simulink model "SoftABS_Hyd_RTW"  (R2022a)
settings: Solver=ode1  StartTime=0.0  StopTime=inf  FixedStep=0.001  RelTol=1e-3
PreLoadFcn:
  | vehicle = 'Car'; if ~length(which('cmcmd')), cmenv; end
  | SoftABS_Hyd_RTW_bus
  | SoftABS_Hyd_RTW_params
InitFcn:
  | vehicle = 'Car'; if ~length(which('cmcmd')), cmenv; end
  | SoftABS_Hyd_RTW_bus
  | SoftABS_Hyd_RTW_params
undefined symbols (not defined in the file or in its folder): f_ax, f_slip, sku_HA, sku_off_HA, sku_off_VA, sku_VA, t_Sensor, v_min, Valve_LUTin_HA, Valve_LUTin_VA, ValveIn_LUTout_HA, ValveIn_LUTout_VA, ValveOut_LUTout_HA, ValveOut_LUTout_VA
libraries: CarMaker4SL x23
Description:
  | CarMaker Plug-in Model Target
settings Model: ModifiedByFormat=IPG  Creator=IPG  LastModifiedBy=IPG
settings SolverCC: AlgebraicLoopSolver=TrustRegion
settings DataIOCC: LimitDataPoints=on  SaveFormat=Array  SignalLoggingSaveFormat=ModelDataLogs  ReturnWorkspaceOutputs=off
settings OptimizationCC: ExpressionDepthLimit=2147483647  LifeSpan=inf
settings DebuggingCC: UnderspecifiedInitializationDetection=Classic  MergeDetectMultiDrivingBlocksExec=none  FcnCallInpInsideContextMsg=warning  UnconnectedInputMsg=warning  UnconnectedOutputMsg=warning  UnconnectedLineMsg=warning  StateNameClashWarn=warning  SFUnexpectedBacktrackingDiag=warning  SFNoUnconditionalDefaultTransitionDiag=warning  SFMachineParentedDataDiag=warning  ArithmeticOperatorsInVariantConditions=warning
settings HardwareCC: ProdBitPerPointer=32  ProdBitPerSizeT=32  ProdBitPerPtrDiffT=32  ProdLargestAtomicFloat=None  ProdIntDivRoundTo=Undefined  ProdEndianess=Unspecified  ProdWordSize=32  ProdHWDeviceType=32-bit Generic  TargetHWDeviceType=32-bit Generic  ProdEqTarget=off
settings ModelReferenceCC: PropagateSignalLabelsOutOfModel=off
settings SFSimCC: SimUseLocalCustomCode=off  CustomCodeUndefinedFunction=UseInterfaceOnly
settings RTWCC: Description=CarMaker Plug-in Model Target  SystemTargetFile=CarMaker.tlc  TemplateMakefile=CarMaker_unix-win64.tmf  RTWUseLocalCustomCode=off  DLArmComputeVersion=19.05
settings CodeAppCC: MaxIdLength=63  StateflowObjectComments=on
settings STFCustomTargetCC: ModelReferenceCompliant=off  CodeInterfacePackaging=Reusable function  CPPClassGenCompliant=on  GRTInterface=off  GenerateAllocFcn=on  SystemTargetFile=CarMaker.tlc
settings GRTTargetCC: TargetLangStandard=C89/C90 (ANSI)  ModelReferenceCompliant=off  ParMdlRefBuildCompliant=off  CompOptLevelCompliant=off  ConcurrentExecutionCompliant=off  CombineOutputUpdateFcns=off  MatFileLogging=off  CodeInterfacePackaging=Reusable function  GenerateAllocFcn=on  UseToolchainInfoCompliant=off  ExtModeMexFile=noextcomm
settings ConfigComp: CovMetricSettings=dw  CovSaveCumulativeToWorkspaceVar=on  CovSaveSingleToWorkspaceVar=on  CovExternalEMLEnable=off

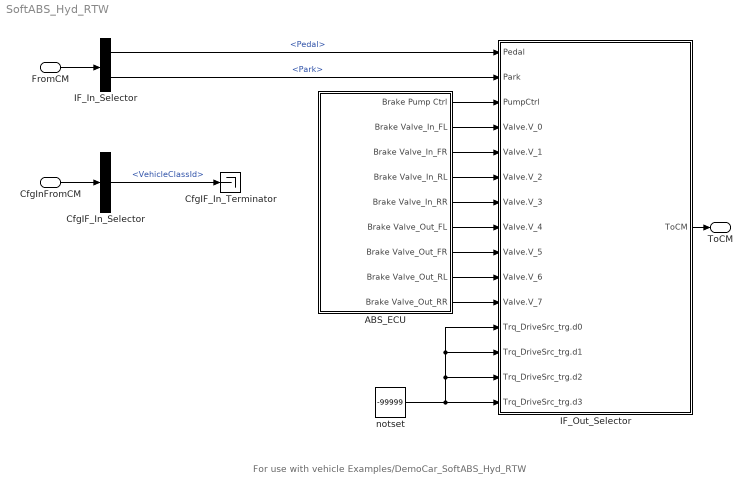
== system SoftABS_Hyd_RTW ==
  note: For use with vehicle Examples/DemoCar_SoftABS_Hyd_RTW
  FromCM : Inport  OutDataTypeStr=Bus: cmHydBrakeControlIn
  CfgInFromCM : Inport  Port=2  OutDataTypeStr=Bus: cmHydBrakeControlCfgIn
  ABS_ECU : Subsystem
  CfgIF_In_Selector : BusSelector  OutputSignals=VehicleClassId
  CfgIF_In_Terminator : Terminator
  IF_In_Selector : BusSelector  OutputSignals=Pedal,Park
  IF_Out_Selector : Subsystem  mask(Signal Selection){}
      mask help: Signal Selection Block
      settings: OpenFcn=cmSignalSelect('SignalSelection_CB',gcb)
  notset : Constant  Value=-99999
  ToCM : Outport  OutDataTypeStr=Bus: cmHydBrakeControlOut  VectorParamsAs1DForOutWhenUnconnected=off
  wires:
  FromCM/1 -> IF_In_Selector/1
  IF_Out_Selector/1(ToCM) -> ToCM/1
  CfgInFromCM/1 -> CfgIF_In_Selector/1
  CfgIF_In_Selector/1 -> CfgIF_In_Terminator/1  "<VehicleClassId>"
  IF_In_Selector/1 -> IF_Out_Selector/1(Pedal)  "<Pedal>"
  IF_In_Selector/2 -> IF_Out_Selector/2(Park)  "<Park>"
  ABS_ECU/9(Brake Valve_Out_RR) -> IF_Out_Selector/11(Valve.V_7)
  ABS_ECU/8(Brake Valve_Out_RL) -> IF_Out_Selector/10(Valve.V_6)
  ABS_ECU/5(Brake Valve_In_RR) -> IF_Out_Selector/7(Valve.V_3)
  ABS_ECU/4(Brake Valve_In_RL) -> IF_Out_Selector/6(Valve.V_2)
  ABS_ECU/3(Brake Valve_In_FR) -> IF_Out_Selector/5(Valve.V_1)
  ABS_ECU/2(Brake Valve_In_FL) -> IF_Out_Selector/4(Valve.V_0)
  ABS_ECU/1(Brake Pump Ctrl) -> IF_Out_Selector/3(PumpCtrl)
  ABS_ECU/6(Brake Valve_Out_FL) -> IF_Out_Selector/8(Valve.V_4)
  ABS_ECU/7(Brake Valve_Out_FR) -> IF_Out_Selector/9(Valve.V_5)
  notset/1 -> IF_Out_Selector/15(Trq_DriveSrc_trg.d3), IF_Out_Selector/14(Trq_DriveSrc_trg.d2), IF_Out_Selector/13(Trq_DriveSrc_trg.d1), IF_Out_Selector/12(Trq_DriveSrc_trg.d0)

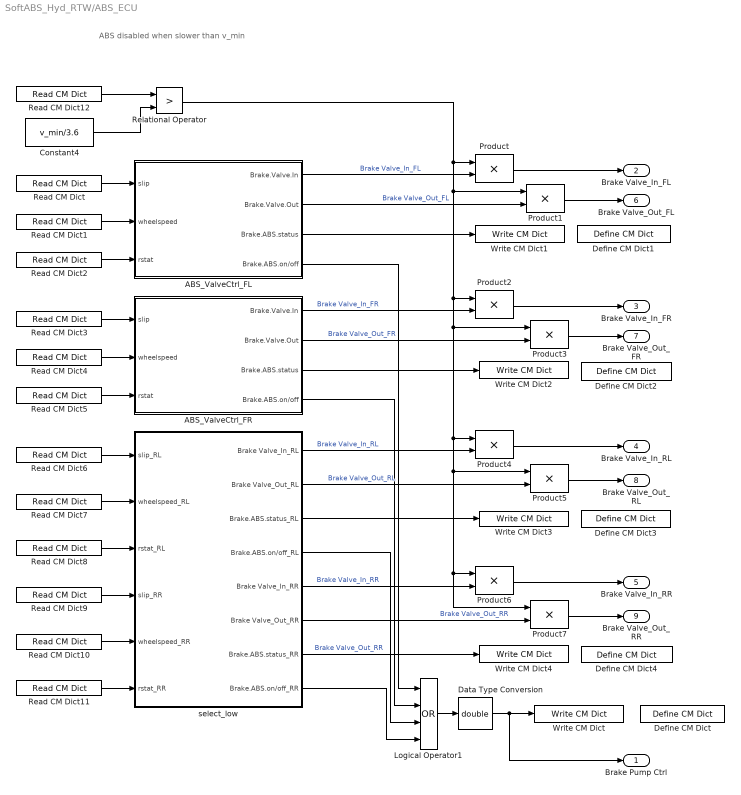
== system SoftABS_Hyd_RTW/ABS_ECU ==
  note: ABS disabled when slower than v_min
  ABS_ValveCtrl_FL : Subsystem
  ABS_ValveCtrl_FR : Subsystem
  Constant4 : Constant  Value=v_min/3.6
  Data Type Conversion : DataTypeConversion  OutDataTypeStr=double  SaturateOnIntegerOverflow=off  RndMeth=Floor
  Define CM Dict : CarMaker4SL/Define CM Dict  xname=ABS.actv  xmono=off  xtype=UChar  xdvaplace=None  xnstates=2  xfirststate=0  xinitial=0
  Define CM Dict1 : CarMaker4SL/Define CM Dict  xname=ABS.Status_FL  xmono=off  xtype=Char  xdvaplace=None  xnstates=4  xfirststate=0  xinitial=0
  Define CM Dict2 : CarMaker4SL/Define CM Dict  xname=ABS.Status_FR  xmono=off  xtype=Char  xdvaplace=None  xnstates=4  xfirststate=0  xinitial=0
  Define CM Dict3 : CarMaker4SL/Define CM Dict  xname=ABS.Status_RL  xmono=off  xtype=Char  xdvaplace=None  xnstates=4  xfirststate=0  xinitial=0
  Define CM Dict4 : CarMaker4SL/Define CM Dict  xname=ABS.Status_RR  xmono=off  xtype=Char  xdvaplace=None  xnstates=4  xfirststate=0  xinitial=0
  Logical Operator1 : Logic  Operator=OR  Inputs=4  AllPortsSameDT=off  OutDataTypeStr=fixdt(1,16)
  Product{,1..7} (8 alike) : Product  OutDataTypeStr=double  SaturateOnIntegerOverflow=on
  Read CM Dict : CarMaker4SL/Read CM Dict  xname=Car.LongSlipFL  xsync=off  xstime=Continuous
  Read CM Dict1 : CarMaker4SL/Read CM Dict  xname=Car.WheelSpd_FL  xsync=off  xstime=Continuous
  Read CM Dict10 : CarMaker4SL/Read CM Dict  xname=Car.WheelSpd_RR  xsync=off  xstime=Continuous
  Read CM Dict11 : CarMaker4SL/Read CM Dict  xname=Car.WRR.Radius  xsync=off  xstime=Continuous
  Read CM Dict12 : CarMaker4SL/Read CM Dict  xname=Car.v  xsync=off  xstime=Continuous
  Read CM Dict2 : CarMaker4SL/Read CM Dict  xname=Car.WFL.Radius  xsync=off  xstime=Continuous
  Read CM Dict3 : CarMaker4SL/Read CM Dict  xname=Car.LongSlipFR  xsync=off  xstime=Continuous
  Read CM Dict4 : CarMaker4SL/Read CM Dict  xname=Car.WheelSpd_FR  xsync=off  xstime=Continuous
  Read CM Dict5 : CarMaker4SL/Read CM Dict  xname=Car.WFR.Radius  xsync=off  xstime=Continuous
  Read CM Dict6 : CarMaker4SL/Read CM Dict  xname=Car.LongSlipRL  xsync=off  xstime=Continuous
  Read CM Dict7 : CarMaker4SL/Read CM Dict  xname=Car.WheelSpd_RL  xsync=off  xstime=Continuous
  Read CM Dict8 : CarMaker4SL/Read CM Dict  xname=Car.WRL.Radius  xsync=off  xstime=Continuous
  Read CM Dict9 : CarMaker4SL/Read CM Dict  xname=Car.LongSlipRR  xsync=off  xstime=Continuous
  Relational Operator : RelationalOperator  Operator=>  InputSameDT=off
  Write CM Dict : CarMaker4SL/Write CM Dict  xname=ABS.actv  xsync=off
  Write CM Dict1 : CarMaker4SL/Write CM Dict  xname=ABS.Status_FL  xsync=off
  Write CM Dict2 : CarMaker4SL/Write CM Dict  xname=ABS.Status_FR  xsync=off
  Write CM Dict3 : CarMaker4SL/Write CM Dict  xname=ABS.Status_RL  xsync=off
  Write CM Dict4 : CarMaker4SL/Write CM Dict  xname=ABS.Status_RR  xsync=off
  select_low : Subsystem
  Brake Pump Ctrl : Outport  VectorParamsAs1DForOutWhenUnconnected=off
  Brake Valve_In_FL : Outport  Port=2  VectorParamsAs1DForOutWhenUnconnected=off
  Brake Valve_In_FR : Outport  Port=3  VectorParamsAs1DForOutWhenUnconnected=off
  Brake Valve_In_RL : Outport  Port=4  VectorParamsAs1DForOutWhenUnconnected=off
  Brake Valve_In_RR : Outport  Port=5  VectorParamsAs1DForOutWhenUnconnected=off
  Brake Valve_Out_FL : Outport  Port=6  VectorParamsAs1DForOutWhenUnconnected=off
  Brake Valve_Out_FR : Outport  Port=7  VectorParamsAs1DForOutWhenUnconnected=off
  Brake Valve_Out_RL : Outport  Port=8  VectorParamsAs1DForOutWhenUnconnected=off
  Brake Valve_Out_RR : Outport  Port=9  VectorParamsAs1DForOutWhenUnconnected=off
  wires:
  Product/1 -> Brake Valve_In_FL/1
  Product1/1 -> Brake Valve_Out_FL/1
  Product2/1 -> Brake Valve_In_FR/1
  Product3/1 -> Brake Valve_Out_FR/1
  Product4/1 -> Brake Valve_In_RL/1
  Product5/1 -> Brake Valve_Out_RL/1
  Product6/1 -> Brake Valve_In_RR/1
  Product7/1 -> Brake Valve_Out_RR/1
  select_low/6(Brake Valve_Out_RR) -> Product7/2  "Brake Valve_Out_RR"
  select_low/5(Brake Valve_In_RR) -> Product6/2  "Brake Valve_In_RR"
  select_low/2(Brake Valve_Out_RL) -> Product5/2  "Brake Valve_Out_RL"
  select_low/1(Brake Valve_In_RL) -> Product4/2  "Brake Valve_In_RL"
  ABS_ValveCtrl_FR/2(Brake.Valve.Out) -> Product3/2  "Brake Valve_Out_FR"
  ABS_ValveCtrl_FR/1(Brake.Valve.In) -> Product2/2  "Brake Valve_In_FR"
  ABS_ValveCtrl_FL/2(Brake.Valve.Out) -> Product1/2  "Brake Valve_Out_FL"
  ABS_ValveCtrl_FL/1(Brake.Valve.In) -> Product/2  "Brake Valve_In_FL"
  Relational Operator/1 -> Product1/1, Product2/1, Product3/1, Product4/1, Product5/1, Product6/1, Product7/1, Product/1
  Constant4/1 -> Relational Operator/2
  Read CM Dict12/1 -> Relational Operator/1
  select_low/8(Brake.ABS.on/off_RR) -> Logical Operator1/4
  select_low/4(Brake.ABS.on/off_RL) -> Logical Operator1/3
  ABS_ValveCtrl_FR/4(Brake.ABS.on/off) -> Logical Operator1/2
  ABS_ValveCtrl_FL/4(Brake.ABS.on/off) -> Logical Operator1/1
  Logical Operator1/1 -> Data Type Conversion/1
  ABS_ValveCtrl_FR/3(Brake.ABS.status) -> Write CM Dict2/1
  select_low/3(Brake.ABS.status_RL) -> Write CM Dict3/1
  ABS_ValveCtrl_FL/3(Brake.ABS.status) -> Write CM Dict1/1
  select_low/7(Brake.ABS.status_RR) -> Write CM Dict4/1  "Brake Valve_Out_RR"
  Read CM Dict11/1 -> select_low/6(rstat_RR)
  Read CM Dict10/1 -> select_low/5(wheelspeed_RR)
  Read CM Dict9/1 -> select_low/4(slip_RR)
  Read CM Dict8/1 -> select_low/3(rstat_RL)
  Read CM Dict7/1 -> select_low/2(wheelspeed_RL)
  Read CM Dict6/1 -> select_low/1(slip_RL)
  Read CM Dict5/1 -> ABS_ValveCtrl_FR/3(rstat)
  Read CM Dict4/1 -> ABS_ValveCtrl_FR/2(wheelspeed)
  Read CM Dict3/1 -> ABS_ValveCtrl_FR/1(slip)
  Read CM Dict2/1 -> ABS_ValveCtrl_FL/3(rstat)
  Read CM Dict1/1 -> ABS_ValveCtrl_FL/2(wheelspeed)
  Read CM Dict/1 -> ABS_ValveCtrl_FL/1(slip)
  Data Type Conversion/1 -> Write CM Dict/1, Brake Pump Ctrl/1

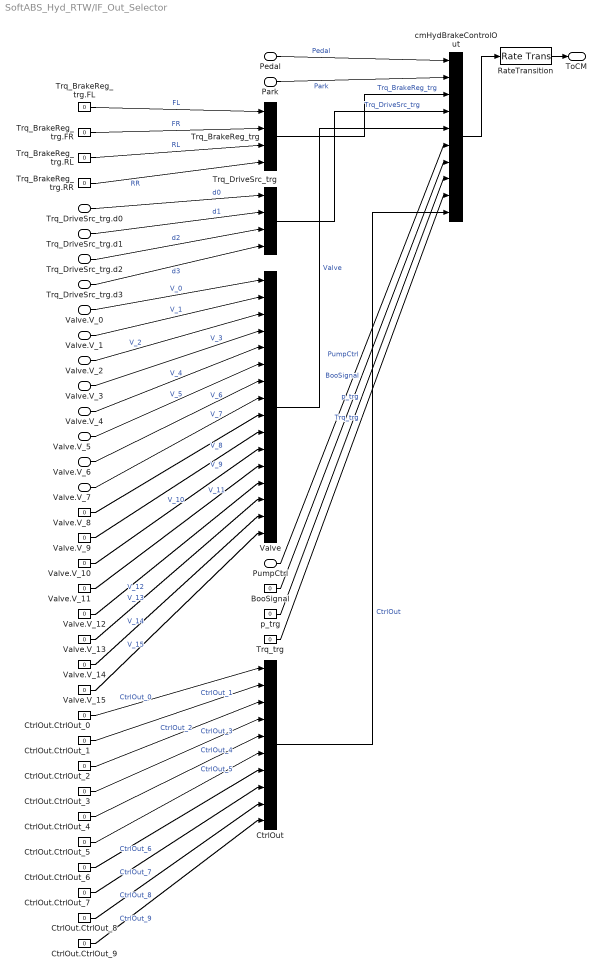
== system SoftABS_Hyd_RTW/IF_Out_Selector ==
  Pedal : Inport
  Park : Inport  Port=2
  PumpCtrl : Inport  Port=3
  Valve.V_0 : Inport  Port=4
  Valve.V_1 : Inport  Port=5
  Valve.V_2 : Inport  Port=6
  Valve.V_3 : Inport  Port=7
  Valve.V_4 : Inport  Port=8
  Valve.V_5 : Inport  Port=9
  Valve.V_6 : Inport  Port=10
  Valve.V_7 : Inport  Port=11
  Trq_DriveSrc_trg.d0 : Inport  Port=12
  Trq_DriveSrc_trg.d1 : Inport  Port=13
  Trq_DriveSrc_trg.d2 : Inport  Port=14
  Trq_DriveSrc_trg.d3 : Inport  Port=15
  BooSignal : Constant  Value=0
  CtrlOut : BusCreator  Inputs=10
  CtrlOut.CtrlOut_{0..9} (10 alike) : Constant  Value=0
  RateTransition : RateTransition  OutPortSampleTime=str2num(get_param(bdroot,'FixedStep'))
  Trq_BrakeReg_trg : BusCreator  Inputs=4
  Trq_BrakeReg_trg.FL : Constant  Value=0
  Trq_BrakeReg_trg.FR : Constant  Value=0
  Trq_BrakeReg_trg.RL : Constant  Value=0
  Trq_BrakeReg_trg.RR : Constant  Value=0
  Trq_DriveSrc_trg : BusCreator  Inputs=4
  Trq_trg : Constant  Value=0
  Valve : BusCreator  Inputs=16
  Valve.V_{8..15} (8 alike) : Constant  Value=0
  cmHydBrakeControlOut : BusCreator  Inputs=10
  p_trg : Constant  Value=0
  ToCM : Outport
  wires:
  RateTransition/1 -> ToCM/1
  cmHydBrakeControlOut/1 -> RateTransition/1
  Trq_BrakeReg_trg/1 -> cmHydBrakeControlOut/3  "Trq_BrakeReg_trg"
  Trq_BrakeReg_trg.FL/1 -> Trq_BrakeReg_trg/1  "FL"
  Trq_BrakeReg_trg.FR/1 -> Trq_BrakeReg_trg/2  "FR"
  Trq_BrakeReg_trg.RL/1 -> Trq_BrakeReg_trg/3  "RL"
  Trq_BrakeReg_trg.RR/1 -> Trq_BrakeReg_trg/4  "RR"
  Trq_DriveSrc_trg/1 -> cmHydBrakeControlOut/4  "Trq_DriveSrc_trg"
  Valve/1 -> cmHydBrakeControlOut/5  "Valve"
  Valve.V_8/1 -> Valve/9  "V_8"
  Valve.V_9/1 -> Valve/10  "V_9"
  Valve.V_10/1 -> Valve/11  "V_10"
  Valve.V_11/1 -> Valve/12  "V_11"
  Valve.V_12/1 -> Valve/13  "V_12"
  Valve.V_13/1 -> Valve/14  "V_13"
  Valve.V_14/1 -> Valve/15  "V_14"
  Valve.V_15/1 -> Valve/16  "V_15"
  BooSignal/1 -> cmHydBrakeControlOut/7  "BooSignal"
  p_trg/1 -> cmHydBrakeControlOut/8  "p_trg"
  Trq_trg/1 -> cmHydBrakeControlOut/9  "Trq_trg"
  CtrlOut/1 -> cmHydBrakeControlOut/10  "CtrlOut"
  CtrlOut.CtrlOut_0/1 -> CtrlOut/1  "CtrlOut_0"
  CtrlOut.CtrlOut_1/1 -> CtrlOut/2  "CtrlOut_1"
  CtrlOut.CtrlOut_2/1 -> CtrlOut/3  "CtrlOut_2"
  CtrlOut.CtrlOut_3/1 -> CtrlOut/4  "CtrlOut_3"
  CtrlOut.CtrlOut_4/1 -> CtrlOut/5  "CtrlOut_4"
  CtrlOut.CtrlOut_5/1 -> CtrlOut/6  "CtrlOut_5"
  CtrlOut.CtrlOut_6/1 -> CtrlOut/7  "CtrlOut_6"
  CtrlOut.CtrlOut_7/1 -> CtrlOut/8  "CtrlOut_7"
  CtrlOut.CtrlOut_8/1 -> CtrlOut/9  "CtrlOut_8"
  CtrlOut.CtrlOut_9/1 -> CtrlOut/10  "CtrlOut_9"
  Pedal/1 -> cmHydBrakeControlOut/1  "Pedal"
  Park/1 -> cmHydBrakeControlOut/2  "Park"
  PumpCtrl/1 -> cmHydBrakeControlOut/6  "PumpCtrl"
  Valve.V_0/1 -> Valve/1  "V_0"
  Valve.V_1/1 -> Valve/2  "V_1"
  Valve.V_2/1 -> Valve/3  "V_2"
  Valve.V_3/1 -> Valve/4  "V_3"
  Valve.V_4/1 -> Valve/5  "V_4"
  Valve.V_5/1 -> Valve/6  "V_5"
  Valve.V_6/1 -> Valve/7  "V_6"
  Valve.V_7/1 -> Valve/8  "V_7"
  Trq_DriveSrc_trg.d0/1 -> Trq_DriveSrc_trg/1  "d0"
  Trq_DriveSrc_trg.d1/1 -> Trq_DriveSrc_trg/2  "d1"
  Trq_DriveSrc_trg.d2/1 -> Trq_DriveSrc_trg/3  "d2"
  Trq_DriveSrc_trg.d3/1 -> Trq_DriveSrc_trg/4  "d3"

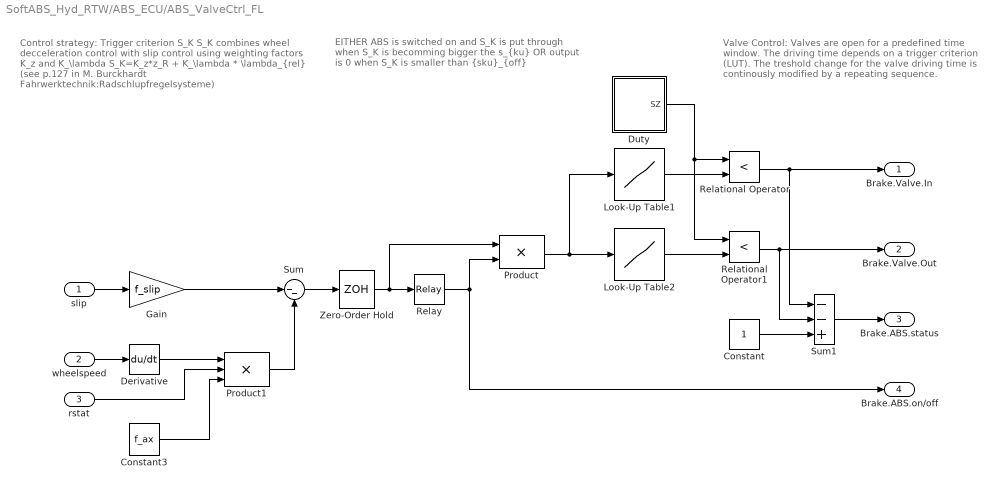
== system SoftABS_Hyd_RTW/ABS_ECU/ABS_ValveCtrl_FL ==
  note: EITHER ABS is switched on and  S_K is put through
      |  when S_K is becomming bigger the s_{ku}
      | OR output is 0 when S_K is smaller than {sku}_{off}
  note: Control strategy: Trigger criterion S_K
      | S_K combines wheel decceleration control with slip control
      | using weighting factors  K_z and K_\lambda
      | S_K=K_z*z_R + K_\lambda * \lambda_{rel}
      | (see p.127 in M. Burckhardt
      | Fahrwerktechnik:Radschlupfregelsysteme)
  note: Valve Control:
      | Valves are open for a predefined time window.
      | The driving time depends on a trigger criterion (LUT).
      | The treshold change for the valve driving time is
      | continously modified by a repeating sequence.
  slip : Inport
  wheelspeed : Inport  Port=2
  rstat : Inport  Port=3
  Constant : Constant
  Constant3 : Constant  Value=f_ax
  Derivative : Derivative
  Duty : Subsystem
  Gain : Gain  Gain=f_slip  SaturateOnIntegerOverflow=on  OutDataTypeStr=Inherit: Same as input  ParamDataTypeStr=Inherit: Same as input
  Look-Up Table1 : Lookup  InputValues=Valve_LUTin_VA  Table=ValveIn_LUTout_VA  LookUpMeth=Interpolation-Use End Values
  Look-Up Table2 : Lookup  InputValues=Valve_LUTin_VA  Table=ValveOut_LUTout_VA  LookUpMeth=Interpolation-Use End Values
  Product : Product  SaturateOnIntegerOverflow=on  OutDataTypeStr=Inherit: Same as first input
  Product1 : Product  Inputs=3  InputSameDT=on  SaturateOnIntegerOverflow=on  OutDataTypeStr=Inherit: Same as first input
  Relational Operator : RelationalOperator  Operator=<  SampleTime=0.001  InputSameDT=off
  Relational Operator1 : RelationalOperator  Operator=<  SampleTime=0.001  InputSameDT=off
  Relay : Relay  OnSwitchValue=sku_VA  OffSwitchValue=sku_off_VA
  Sum : Sum  Inputs=|--  InputSameDT=on  SaturateOnIntegerOverflow=on  OutDataTypeStr=Inherit: Same as first input
  Sum1 : Sum  Inputs=--+  SaturateOnIntegerOverflow=on
  Zero-Order Hold : ZeroOrderHold  SampleTime=t_Sensor
  Brake.Valve.In : Outport  VectorParamsAs1DForOutWhenUnconnected=off
  Brake.Valve.Out : Outport  Port=2  VectorParamsAs1DForOutWhenUnconnected=off
  Brake.ABS.status : Outport  Port=3  VectorParamsAs1DForOutWhenUnconnected=off
  Brake.ABS.on/off : Outport  Port=4  VectorParamsAs1DForOutWhenUnconnected=off
  wires:
  Derivative/1 -> Product1/1
  Gain/1 -> Sum/1
  Product1/1 -> Sum/2
  slip/1 -> Gain/1
  wheelspeed/1 -> Derivative/1
  rstat/1 -> Product1/2
  Constant3/1 -> Product1/3
  Relational Operator/1 -> Brake.Valve.In/1, Sum1/1
  Relational Operator1/1 -> Brake.Valve.Out/1, Sum1/2
  Constant/1 -> Sum1/3
  Sum1/1 -> Brake.ABS.status/1
  Sum/1 -> Zero-Order Hold/1
  Product/1 -> Look-Up Table1/1, Look-Up Table2/1
  Duty/1(SZ) -> Relational Operator1/1, Relational Operator/1
  Look-Up Table1/1 -> Relational Operator/2
  Look-Up Table2/1 -> Relational Operator1/2
  Relay/1 -> Product/2, Brake.ABS.on/off/1
  Zero-Order Hold/1 -> Relay/1, Product/1

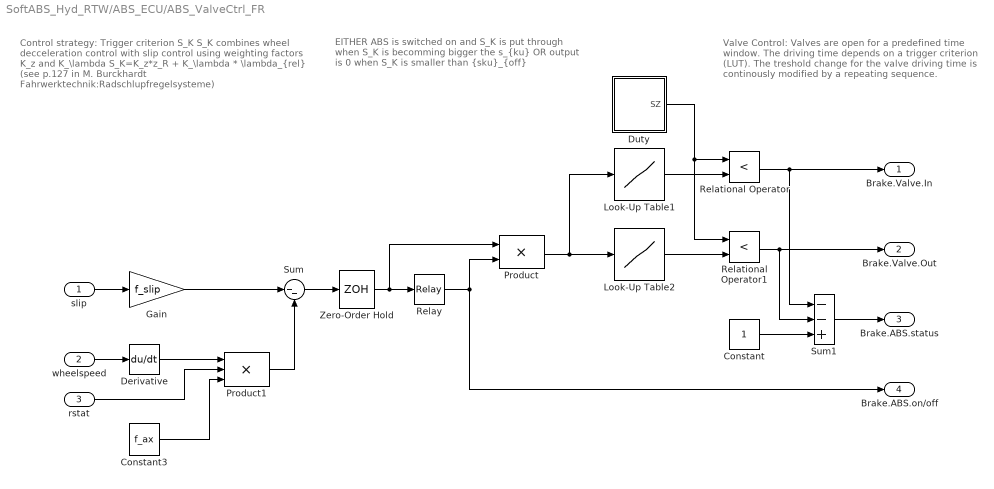
== system SoftABS_Hyd_RTW/ABS_ECU/ABS_ValveCtrl_FR ==
  note: EITHER ABS is switched on and  S_K is put through
      |  when S_K is becomming bigger the s_{ku}
      | OR output is 0 when S_K is smaller than {sku}_{off}
  note: Control strategy: Trigger criterion S_K
      | S_K combines wheel decceleration control with slip control
      | using weighting factors  K_z and K_\lambda
      | S_K=K_z*z_R + K_\lambda * \lambda_{rel}
      | (see p.127 in M. Burckhardt
      | Fahrwerktechnik:Radschlupfregelsysteme)
  note: Valve Control:
      | Valves are open for a predefined time window.
      | The driving time depends on a trigger criterion (LUT).
      | The treshold change for the valve driving time is
      | continously modified by a repeating sequence.
  slip : Inport
  wheelspeed : Inport  Port=2
  rstat : Inport  Port=3
  Constant : Constant
  Constant3 : Constant  Value=f_ax
  Derivative : Derivative
  Duty : Subsystem
  Gain : Gain  Gain=f_slip  SaturateOnIntegerOverflow=on  OutDataTypeStr=Inherit: Same as input  ParamDataTypeStr=Inherit: Same as input
  Look-Up Table1 : Lookup  InputValues=Valve_LUTin_VA  Table=ValveIn_LUTout_VA  LookUpMeth=Interpolation-Use End Values
  Look-Up Table2 : Lookup  InputValues=Valve_LUTin_VA  Table=ValveOut_LUTout_VA  LookUpMeth=Interpolation-Use End Values
  Product : Product  SaturateOnIntegerOverflow=on  OutDataTypeStr=Inherit: Same as first input
  Product1 : Product  Inputs=3  InputSameDT=on  SaturateOnIntegerOverflow=on  OutDataTypeStr=Inherit: Same as first input
  Relational Operator : RelationalOperator  Operator=<  SampleTime=0.001  InputSameDT=off
  Relational Operator1 : RelationalOperator  Operator=<  SampleTime=0.001  InputSameDT=off
  Relay : Relay  OnSwitchValue=sku_VA  OffSwitchValue=sku_off_VA
  Sum : Sum  Inputs=|--  InputSameDT=on  SaturateOnIntegerOverflow=on  OutDataTypeStr=Inherit: Same as first input
  Sum1 : Sum  Inputs=--+  SaturateOnIntegerOverflow=on
  Zero-Order Hold : ZeroOrderHold  SampleTime=t_Sensor
  Brake.Valve.In : Outport  VectorParamsAs1DForOutWhenUnconnected=off
  Brake.Valve.Out : Outport  Port=2  VectorParamsAs1DForOutWhenUnconnected=off
  Brake.ABS.status : Outport  Port=3  VectorParamsAs1DForOutWhenUnconnected=off
  Brake.ABS.on/off : Outport  Port=4  VectorParamsAs1DForOutWhenUnconnected=off
  wires:
  Derivative/1 -> Product1/1
  Gain/1 -> Sum/1
  Product1/1 -> Sum/2
  slip/1 -> Gain/1
  wheelspeed/1 -> Derivative/1
  rstat/1 -> Product1/2
  Constant3/1 -> Product1/3
  Relational Operator/1 -> Brake.Valve.In/1, Sum1/1
  Relational Operator1/1 -> Brake.Valve.Out/1, Sum1/2
  Constant/1 -> Sum1/3
  Sum1/1 -> Brake.ABS.status/1
  Sum/1 -> Zero-Order Hold/1
  Product/1 -> Look-Up Table1/1, Look-Up Table2/1
  Duty/1(SZ) -> Relational Operator1/1, Relational Operator/1
  Look-Up Table1/1 -> Relational Operator/2
  Look-Up Table2/1 -> Relational Operator1/2
  Relay/1 -> Product/2, Brake.ABS.on/off/1
  Zero-Order Hold/1 -> Relay/1, Product/1

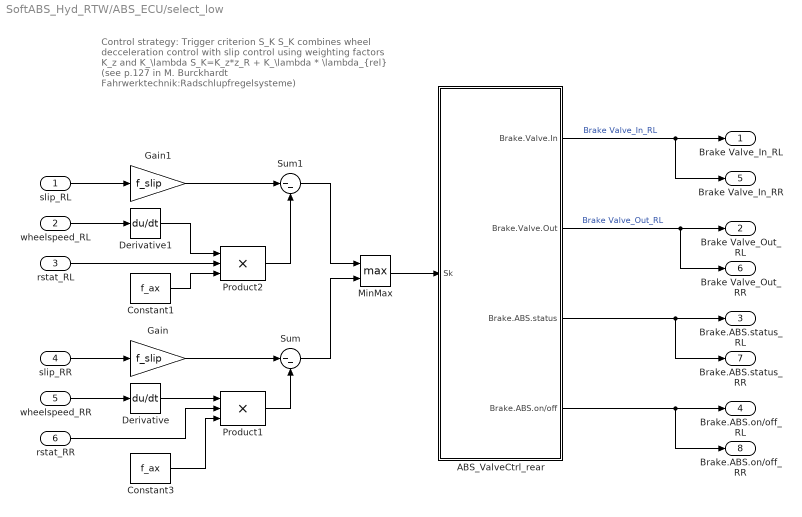
== system SoftABS_Hyd_RTW/ABS_ECU/select_low ==
  note: Control strategy: Trigger criterion S_K
      | S_K combines wheel decceleration control with slip control
      | using weighting factors  K_z and K_\lambda
      | S_K=K_z*z_R + K_\lambda * \lambda_{rel}
      | (see p.127 in M. Burckhardt
      | Fahrwerktechnik:Radschlupfregelsysteme)
  slip_RL : Inport
  wheelspeed_RL : Inport  Port=2
  rstat_RL : Inport  Port=3
  slip_RR : Inport  Port=4
  wheelspeed_RR : Inport  Port=5
  rstat_RR : Inport  Port=6
  ABS_ValveCtrl_rear : Subsystem
  Constant1 : Constant  Value=f_ax
  Constant3 : Constant  Value=f_ax
  Derivative : Derivative
  Derivative1 : Derivative
  Gain : Gain  Gain=f_slip  SaturateOnIntegerOverflow=on  OutDataTypeStr=Inherit: Same as input  ParamDataTypeStr=Inherit: Same as input
  Gain1 : Gain  Gain=f_slip  SaturateOnIntegerOverflow=on  OutDataTypeStr=Inherit: Same as input  ParamDataTypeStr=Inherit: Same as input
  MinMax : MinMax  Function=max  Inputs=2  InputSameDT=on  SaturateOnIntegerOverflow=on
  Product1 : Product  Inputs=3  InputSameDT=on  SaturateOnIntegerOverflow=on  OutDataTypeStr=Inherit: Same as first input
  Product2 : Product  Inputs=3  InputSameDT=on  SaturateOnIntegerOverflow=on  OutDataTypeStr=Inherit: Same as first input
  Sum : Sum  Inputs=|--  InputSameDT=on  SaturateOnIntegerOverflow=on  OutDataTypeStr=Inherit: Same as first input
  Sum1 : Sum  Inputs=|--  InputSameDT=on  SaturateOnIntegerOverflow=on  OutDataTypeStr=Inherit: Same as first input
  Brake Valve_In_RL : Outport  VectorParamsAs1DForOutWhenUnconnected=off
  Brake Valve_Out_RL : Outport  Port=2  VectorParamsAs1DForOutWhenUnconnected=off
  Brake.ABS.status_RL : Outport  Port=3  VectorParamsAs1DForOutWhenUnconnected=off
  Brake.ABS.on/off_RL : Outport  Port=4  VectorParamsAs1DForOutWhenUnconnected=off
  Brake Valve_In_RR : Outport  Port=5  VectorParamsAs1DForOutWhenUnconnected=off
  Brake Valve_Out_RR : Outport  Port=6  VectorParamsAs1DForOutWhenUnconnected=off
  Brake.ABS.status_RR : Outport  Port=7  VectorParamsAs1DForOutWhenUnconnected=off
  Brake.ABS.on/off_RR : Outport  Port=8  VectorParamsAs1DForOutWhenUnconnected=off
  wires:
  rstat_RR/1 -> Product1/2
  wheelspeed_RR/1 -> Derivative/1
  slip_RR/1 -> Gain/1
  ABS_ValveCtrl_rear/4(Brake.ABS.on/off) -> Brake.ABS.on/off_RL/1, Brake.ABS.on/off_RR/1
  ABS_ValveCtrl_rear/3(Brake.ABS.status) -> Brake.ABS.status_RL/1, Brake.ABS.status_RR/1
  ABS_ValveCtrl_rear/2(Brake.Valve.Out) -> Brake Valve_Out_RL/1, Brake Valve_Out_RR/1  "Brake Valve_Out_RL"
  ABS_ValveCtrl_rear/1(Brake.Valve.In) -> Brake Valve_In_RL/1, Brake Valve_In_RR/1  "Brake Valve_In_RL"
  Derivative/1 -> Product1/1
  Gain/1 -> Sum/1
  Product1/1 -> Sum/2
  Constant3/1 -> Product1/3
  Derivative1/1 -> Product2/1
  Gain1/1 -> Sum1/1
  Product2/1 -> Sum1/2
  Constant1/1 -> Product2/3
  slip_RL/1 -> Gain1/1
  wheelspeed_RL/1 -> Derivative1/1
  rstat_RL/1 -> Product2/2
  Sum1/1 -> MinMax/1
  Sum/1 -> MinMax/2
  MinMax/1 -> ABS_ValveCtrl_rear/1(Sk)

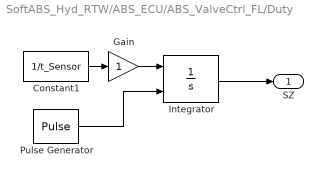
== system SoftABS_Hyd_RTW/ABS_ECU/ABS_ValveCtrl_FL/Duty ==
  Constant1 : Constant  Value=1/t_Sensor
  Gain : Gain
  Integrator : Integrator  ExternalReset=either
  Pulse Generator : DiscretePulseGenerator  PulseType=Time based  Period=t_Sensor*2  PulseWidth=50
  SZ : Outport  VectorParamsAs1DForOutWhenUnconnected=off
  wires:
  Constant1/1 -> Gain/1
  Pulse Generator/1 -> Integrator/2
  Integrator/1 -> SZ/1
  Gain/1 -> Integrator/1

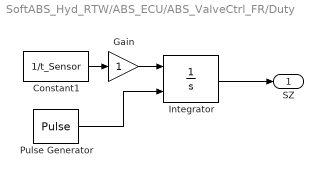
== system SoftABS_Hyd_RTW/ABS_ECU/ABS_ValveCtrl_FR/Duty ==
  Constant1 : Constant  Value=1/t_Sensor
  Gain : Gain
  Integrator : Integrator  ExternalReset=either
  Pulse Generator : DiscretePulseGenerator  PulseType=Time based  Period=t_Sensor*2  PulseWidth=50
  SZ : Outport  VectorParamsAs1DForOutWhenUnconnected=off
  wires:
  Constant1/1 -> Gain/1
  Pulse Generator/1 -> Integrator/2
  Integrator/1 -> SZ/1
  Gain/1 -> Integrator/1

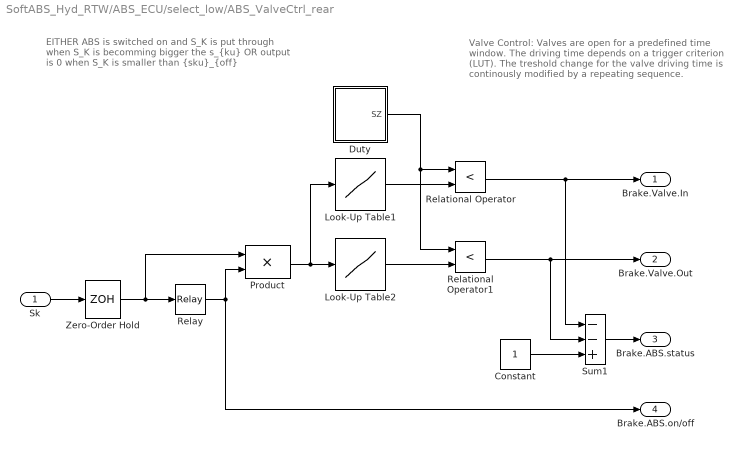
== system SoftABS_Hyd_RTW/ABS_ECU/select_low/ABS_ValveCtrl_rear ==
  note: EITHER ABS is switched on and  S_K is put through
      |  when S_K is becomming bigger the s_{ku}
      | OR output is 0 when S_K is smaller than {sku}_{off}
  note: Valve Control:
      | Valves are open for a predefined time window.
      | The driving time depends on a trigger criterion (LUT).
      | The treshold change for the valve driving time is
      | continously modified by a repeating sequence.
  Sk : Inport
  Constant : Constant
  Duty : Subsystem
  Look-Up Table1 : Lookup  InputValues=Valve_LUTin_HA  Table=ValveIn_LUTout_HA  LookUpMeth=Interpolation-Use End Values
  Look-Up Table2 : Lookup  InputValues=Valve_LUTin_HA  Table=ValveOut_LUTout_HA  LookUpMeth=Interpolation-Use End Values
  Product : Product  SaturateOnIntegerOverflow=on  OutDataTypeStr=Inherit: Same as first input
  Relational Operator : RelationalOperator  Operator=<  SampleTime=0.001  InputSameDT=off
  Relational Operator1 : RelationalOperator  Operator=<  SampleTime=0.001  InputSameDT=off
  Relay : Relay  OnSwitchValue=sku_HA  OffSwitchValue=sku_off_HA
  Sum1 : Sum  Inputs=--+  SaturateOnIntegerOverflow=on
  Zero-Order Hold : ZeroOrderHold  SampleTime=t_Sensor
  Brake.Valve.In : Outport  VectorParamsAs1DForOutWhenUnconnected=off
  Brake.Valve.Out : Outport  Port=2  VectorParamsAs1DForOutWhenUnconnected=off
  Brake.ABS.status : Outport  Port=3  VectorParamsAs1DForOutWhenUnconnected=off
  Brake.ABS.on/off : Outport  Port=4  VectorParamsAs1DForOutWhenUnconnected=off
  wires:
  Relational Operator/1 -> Brake.Valve.In/1, Sum1/1
  Relational Operator1/1 -> Brake.Valve.Out/1, Sum1/2
  Constant/1 -> Sum1/3
  Sum1/1 -> Brake.ABS.status/1
  Duty/1(SZ) -> Relational Operator/1, Relational Operator1/1
  Look-Up Table1/1 -> Relational Operator/2
  Look-Up Table2/1 -> Relational Operator1/2
  Zero-Order Hold/1 -> Relay/1, Product/1
  Relay/1 -> Product/2, Brake.ABS.on/off/1
  Product/1 -> Look-Up Table1/1, Look-Up Table2/1
  Sk/1 -> Zero-Order Hold/1

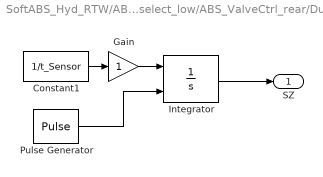
== system SoftABS_Hyd_RTW/ABS_ECU/select_low/ABS_ValveCtrl_rear/Duty ==
  Constant1 : Constant  Value=1/t_Sensor
  Gain : Gain
  Integrator : Integrator  ExternalReset=either
  Pulse Generator : DiscretePulseGenerator  PulseType=Time based  Period=t_Sensor*2  PulseWidth=50
  SZ : Outport  VectorParamsAs1DForOutWhenUnconnected=off
  wires:
  Constant1/1 -> Gain/1
  Pulse Generator/1 -> Integrator/2
  Integrator/1 -> SZ/1
  Gain/1 -> Integrator/1
